simulink model "Model_FL_APF_WF_VO"  (R2024b)
settings: Solver=FixedStepAuto  StartTime=0.0  StopTime=150  FixedStep=UAVSampleTime  RelTol=1e-3
undefined symbols (not defined in the file): DroneMass, Gravity, Horizontal_Limits, Horizontal_Res, kD_pos, kD_vel, kI_pos, kI_vel, kP_pos, kP_vel, Lidar, MaxRange, N_filter, TopSpeed, UAV, Vertical_Limits, Vertical_Res, Waypoints
libraries: slpidlib x6, uavsimlib x4, fuzblock x2, robotcorelib x1, uavalgslib x1
(part 2 of 2)

== matlab function Model_FL_APF_WF_VO/LML Indicators/LML_indicators ==
  settings: updateMethod=DISCRETE
  data: APF_pos input; APF_mag output; position input; target input; disp_1s output; t input; disp_3s output; dist2goal output
function [APF_mag, disp_1s, disp_3s, dist2goal] = LML_indicators(APF_pos, position, target, t)

Tmax = 180;

persistent pos_hist
persistent lastSec

if isempty(pos_hist)
    pos_hist = zeros(Tmax+1, 3);
    lastSec  = int32(-1);
end

% APF_mag 
APF_mag = norm(APF_pos(:) - position(:));

% Time and Pos_hist
sec = int32(floor(t));
if sec ~= lastSec && sec >= 0 && sec <= Tmax
    pos_hist(sec+1, :) = position(:).';
    lastSec = sec;
end

% Disp1s
if sec >= 1
    disp_1s = norm(position(:) - pos_hist(sec, :).');
else
    disp_1s = 0;
end

% Disp3s
if sec >= 3
    disp_3s = norm(position(:) - pos_hist(sec-2, :).');
else
    disp_3s = 0;
end

% Dist2goal
dist2goal = norm(target-position);

== matlab function Model_FL_APF_WF_VO/Controller/Attitude Control/Multirotor Acceleration Control ==
  data: acc input; roll output; pitch output; thrust output; yaw input; DroneMass parameter; Gravity parameter
function [roll, pitch, thrust] = accControl(acc, yaw, DroneMass, Gravity)

    xddot = acc(1);
    yddot = acc(2);
    zddot = acc(3);
    
    pitch = atan2((-xddot*cos(yaw)-yddot*sin(yaw)), ( -zddot + Gravity));
    roll = atan2(((-xddot*sin(yaw)+yddot*cos(yaw))*cos(pitch)), (-zddot+Gravity));
    
    roll_limit = 25*pi/180;
    pitch_limit = 25*pi/180;
    
    roll = min(roll_limit, max(-roll_limit, roll));
   
    pitch = min(pitch_limit, max(-pitch_limit, pitch));
    
    thrust = DroneMass*(-zddot+Gravity)/(cos(pitch)*cos(roll));
end

== matlab function Model_FL_APF_WF_VO/Path Planning Data/VOActivator_V5 ==
  settings: updateMethod=DISCRETE
  data: Minima_list input; Minima_count input; position input; Virtuals_list output; flight_mode input; Virtuals_count output; t input
function [Virtuals_list, Virtuals_count] = VOActivator(Minima_list, Minima_count, position, flight_mode, t)

activation_dist = 3;
maxVO = 100;

persistent VO_list
persistent VO_count
persistent next_to_check
persistent was_in_WF

if isempty(VO_list)
    VO_list      = zeros(maxVO, 3);
    VO_count     = 0;
    next_to_check = 1;
    was_in_WF     = false(maxVO, 1);

    % Pass to workspace at least once
    assignin('base', 'finalVOList',  VO_list);
    assignin('base', 'finalVOCount', VO_count);
    
end

% Mark all current unactivated minima as having been in WF
if flight_mode == 2 || flight_mode == 3
    was_in_WF(next_to_check:Minima_count) = true;
end

% Check unactivated minima for activation
for i = next_to_check:Minima_count
    d = norm(position(:) - Minima_list(i,:).');
    if d > activation_dist || (flight_mode == 1 && was_in_WF(i))
        % VO is activated
        %disp("VO Activated at t ="); disp(t);
        VO_count = VO_count + 1;
        VO_list(VO_count, :) = Minima_list(i,:);
        next_to_check = i + 1;
        % Update VO list in workspace
        assignin('base', 'finalVOList',  VO_list);
        assignin('base', 'finalVOCount', VO_count);
    end
end

Virtuals_list  = VO_list;
Virtuals_count = VO_count;

== matlab function Model_FL_APF_WF_VO/CPL Indicators/CPL_Indicators ==
  data: APF_pos input; APF_WF_ang output; WF_pos input; position input; Minima_list input; Minima_count input; cloud input; dist_closest_minima output; angular_coverage output
function [APF_WF_ang, dist_closest_minima, angular_coverage] = CPL_inputs(APF_pos, WF_pos, position, Minima_list, Minima_count, cloud)

% Parameters
max_dist = 10;
n_bins   = 36;

% APF_WF angle
APF_dir    = APF_pos(:) - position(:);
WF_dir     = WF_pos(:)  - position(:);
APF_WF_ang = rad2deg(acos(dot(APF_dir, WF_dir)/max(1e-6,(norm(APF_dir)*norm(WF_dir)))));

% Distance to closest minima
if Minima_count > 0
    diffs = Minima_list(1:Minima_count,:) - position(:).';
    dists = sqrt(sum(diffs.^2, 2));
    dist_closest_minima = min([min(dists(:)), max_dist]);
else
    dist_closest_minima = max_dist;
end

% Angular coverage

bearings = atan2(cloud(:,2), cloud(:,1));
bin_indices = mod(floor(bearings / (2*pi/n_bins)), n_bins) + 1;
bin_indices = max(1, min(n_bins, bin_indices));
bins = false(n_bins, 1);
bins(bin_indices) = true;
angular_coverage = sum(bins) / n_bins;

== matlab function Model_FL_APF_WF_VO/Path Planning Data/GoalReached_V5 ==
  settings: updateMethod=DISCRETE
  data: time input; currentWaypoint output; endSim output; pos input; waypoints input
function [currentWaypoint, endSim] = fcn(time, pos, waypoints)

waypoint_threshold = 0.25;

persistent idx;
persistent numWaypoints;
if isempty(idx)
    idx = 1;
    numWaypoints = size(waypoints, 1);
end

if norm(waypoints(idx,:).' - pos) < waypoint_threshold
    disp('Reached Waypoint');
    disp(idx);
    idx = idx + 1;
end

if idx > numWaypoints
    endSim = 1;
    currentWaypoint = waypoints(end,:).'; % can't have it empty
    disp('Sim ended at t =');
    disp(time);
    return;
end

currentWaypoint = waypoints(idx,:).';
endSim = 0;

== matlab function Model_FL_APF_WF_VO/FL Mode Switcher/FL Switcher ==
  settings: updateMethod=DISCRETE
  data: position input; flight_mode output; goal input; cloud input; APF_pos input; WF_pos input; LML input; CPL input; desired_pos output; Minima_list output; Minima_count output; critPoint_list output; critPoint_count output; t input
function [flight_mode, desired_pos, Minima_list, Minima_count, critPoint_list, critPoint_count] = FL_modeManager(position, goal, cloud, APF_pos, WF_pos, LML, CPL, t)

% Parameters
LML_threshold = 0.8;
CPL_threshold = 0.7;
minimaMax     = 100;
CPmax         = 100;

% Persistent variables
persistent mode
persistent LM_list
persistent LM_count
persistent CP_list
persistent CP_count

if isempty(mode)
    mode    = 1;
    LM_list = zeros(minimaMax, 3);
    LM_count = 0;
    CP_list = zeros(CPmax, 3);
    CP_count = 0;
    assignin('base', 'finalMinimaList',  LM_list);
    assignin('base', 'finalMinimaCount', LM_count);
    assignin('base', 'finalCPList',      CP_list);
    assignin('base', 'finalCPCount',     CP_count);
end

% Default outputs
flight_mode     = mode;
desired_pos     = APF_pos;
Minima_list     = LM_list;
Minima_count    = LM_count;
critPoint_list  = CP_list;
critPoint_count = CP_count;

switch mode

    case 1  % APF mode
        desired_pos = APF_pos;
        if LML > LML_threshold
            %disp('Local Minima Detected at t ='); disp(t);
            LM_count = LM_count + 1;
            LM_list(LM_count, :) = position(:).';
            assignin('base', 'finalMinimaList',  LM_list);
            assignin('base', 'finalMinimaCount', LM_count);
            Minima_list  = LM_list;
            Minima_count = LM_count;
            % Determine Left or Right
            forwardXY    = goal(1:2) - position(1:2);
            cross_z      = forwardXY(1)*cloud(:,2) - cloud(:,1)*forwardXY(2);
            left_points  = sum(cross_z > 0);
            right_points = sum(cross_z < 0);
            if left_points < right_points
                mode = 2;
            else
                mode = 3;
            end
        end
        flight_mode = mode;

    case {2, 3}  % WF mode
        desired_pos = WF_pos;
        if CPL > CPL_threshold
            %disp('Critical Point Detected at t ='); disp(t);
            CP_count = CP_count + 1;
            CP_list(CP_count, :) = position(:).';
            assignin('base', 'finalCPList',  CP_list);
            assignin('base', 'finalCPCount', CP_count);
            critPoint_list  = CP_list;
            critPoint_count = CP_count;
            mode = 1;
        end
        flight_mode = mode;

    otherwise
        desired_pos = APF_pos;
        flight_mode = mode;
end
